simulink model "Robust_design_sinusoidal_validation"  (R2025b)
settings: Solver=VariableStepAuto  StartTime=0.0  StopTime=20  FixedStep=0.001  RelTol=1e-3
undefined symbols (not defined in the file): daq, degs2rpm, den, den_G, drv, Kxi, num, num_G, rdp, rpm2rads, sens, Ts, u_bar_max
settings Model: Creator=Enrico  LastModifiedBy=Enrico
settings DataIOCC: ReturnWorkspaceOutputsName=out_black_box

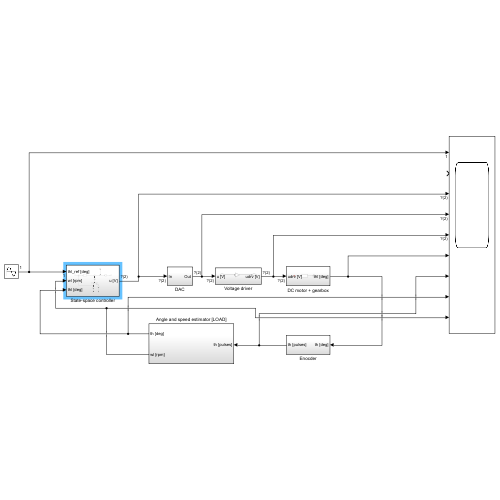
[thumbnail: Simulink's stored preview of the top-level diagram]
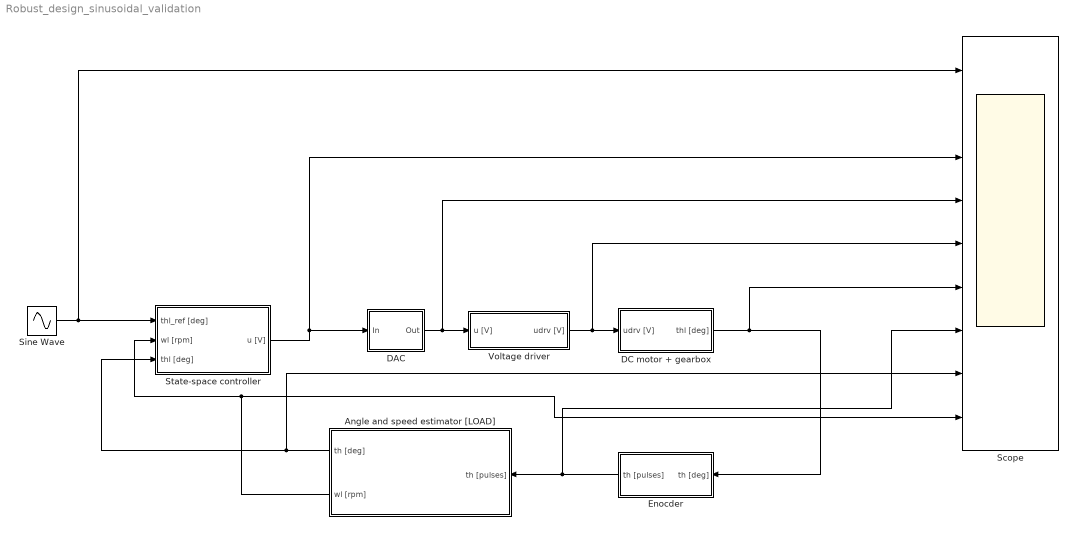
== system Robust_design_sinusoidal_validation ==
  Angle and speed estimator [LOAD] : Subsystem
  DAC : Subsystem
  DC motor + gearbox : Subsystem
  Enocder : Subsystem
  Scope : Scope  NumInputPorts=9
      settings: ActiveDisplayYMinimum=-1.2803910896593547  ActiveDisplayYMaximum=1.2800791059600789
  Sine Wave : Sin  Frequency=2*pi*0.5  SampleTime=0
  State-space controller : Subsystem
  Voltage driver : Subsystem
  wires:
  State-space controller/1(u [V]) -> Scope/3, DAC/1(In)
  DAC/1(Out) -> Scope/4, Voltage driver/1(u [V])
  Sine Wave/1 -> Scope/1, State-space controller/1(thl_ref [deg])
  Enocder/1(th [pulses]) -> Scope/7, Angle and speed estimator [LOAD]/1(th [pulses])
  Voltage driver/1(udrv [V]) -> Scope/5, DC motor + gearbox/1(udrv [V])
  DC motor + gearbox/1(thl [deg]) -> Scope/6, Enocder/1(th [deg])
  Angle and speed estimator [LOAD]/1(th [deg]) -> State-space controller/3(thl [deg]), Scope/8
  Angle and speed estimator [LOAD]/2(wl [rpm]) -> State-space controller/2(wl [rpm]), Scope/9

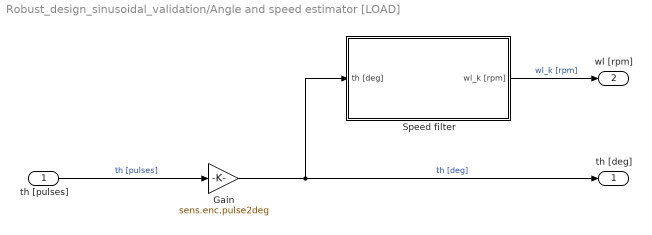
== system Robust_design_sinusoidal_validation/Angle and speed estimator [LOAD] ==
  th [pulses] : Inport
  Gain : Gain  Gain=sens.enc.pulse2deg
  Speed filter : Subsystem
  th [deg] : Outport
  wl [rpm] : Outport  Port=2
  wires:
  Speed filter/1(wl_k [rpm]) -> wl [rpm]/1  "wl_k [rpm]"
  th [pulses]/1 -> Gain/1  "th [pulses]"
  Gain/1 -> Speed filter/1(th [deg]), th [deg]/1  "th [deg]"

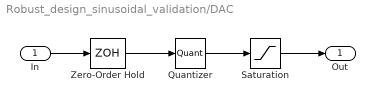
== system Robust_design_sinusoidal_validation/DAC ==
  In : Inport
  Quantizer : Quantizer  QuantizationInterval=daq.dac.q
  Saturation : Saturate  UpperLimit=daq.dac.fs  LowerLimit=-daq.dac.fs
  Zero-Order Hold : ZeroOrderHold  SampleTime=Ts
  Out : Outport
  wires:
  Quantizer/1 -> Saturation/1
  In/1 -> Zero-Order Hold/1
  Zero-Order Hold/1 -> Quantizer/1
  Saturation/1 -> Out/1

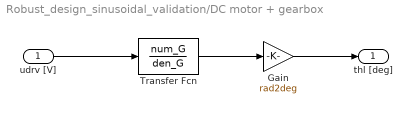
== system Robust_design_sinusoidal_validation/DC motor + gearbox ==
  udrv [V] : Inport
  Gain : Gain  Gain=rad2deg
  Transfer Fcn : TransferFcn  Numerator=num_G  Denominator=den_G
  thl [deg] : Outport
  wires:
  udrv [V]/1 -> Transfer Fcn/1
  Transfer Fcn/1 -> Gain/1
  Gain/1 -> thl [deg]/1

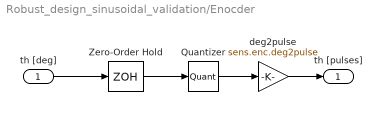
== system Robust_design_sinusoidal_validation/Enocder ==
  th [deg] : Inport
  Quantizer : Quantizer  QuantizationInterval=sens.enc.pulse2deg
  Zero-Order Hold : ZeroOrderHold  SampleTime=Ts
  deg2pulse : Gain  Gain=sens.enc.deg2pulse
  th [pulses] : Outport
  wires:
  Quantizer/1 -> deg2pulse/1
  th [deg]/1 -> Zero-Order Hold/1
  Zero-Order Hold/1 -> Quantizer/1
  deg2pulse/1 -> th [pulses]/1

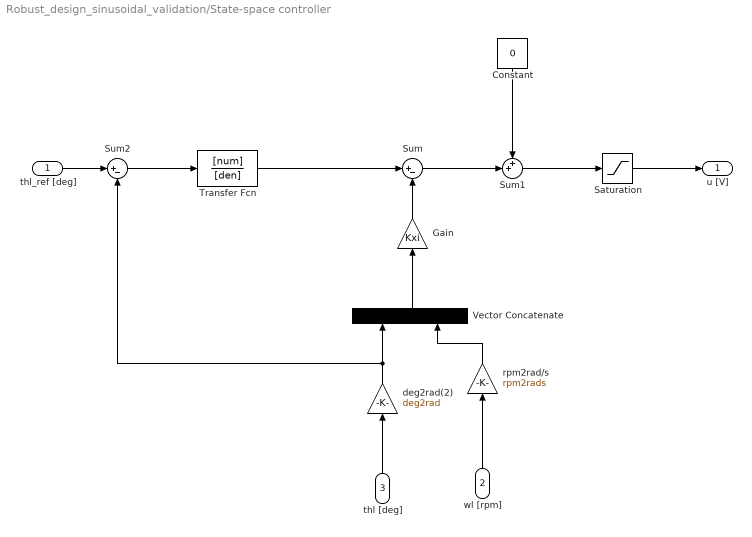
== system Robust_design_sinusoidal_validation/State-space controller ==
  thl_ref [deg] : Inport
  wl [rpm] : Inport  Port=2
  thl [deg] : Inport  Port=3
  Constant : Constant  Value=0
  Gain : Gain  Gain=Kxi
  Saturation : Saturate  UpperLimit=u_bar_max  LowerLimit=-u_bar_max
  Sum : Sum  Inputs=|+-
  Sum1 : Sum  Inputs=++|
  Sum2 : Sum  Inputs=|+-
  Transfer Fcn : TransferFcn  Numerator=[num]  Denominator=[den]
  Vector Concatenate : Concatenate
  deg2rad(2) : Gain  Gain=deg2rad
  rpm2rad/s : Gain  Gain=rpm2rads
  u [V] : Outport
  wires:
  Saturation/1 -> u [V]/1
  Sum/1 -> Sum1/2
  wl [rpm]/1 -> rpm2rad/s/1
  thl [deg]/1 -> deg2rad(2)/1
  deg2rad(2)/1 -> Sum2/2, Vector Concatenate/1
  rpm2rad/s/1 -> Vector Concatenate/2
  Vector Concatenate/1 -> Gain/1
  Gain/1 -> Sum/2
  Sum1/1 -> Saturation/1
  Sum2/1 -> Transfer Fcn/1
  thl_ref [deg]/1 -> Sum2/1
  Transfer Fcn/1 -> Sum/1
  Constant/1 -> Sum1/1

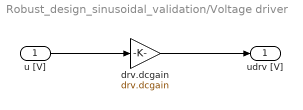
== system Robust_design_sinusoidal_validation/Voltage driver ==
  u [V] : Inport
  drv.dcgain : Gain  Gain=drv.dcgain
  udrv [V] : Outport
  wires:
  u [V]/1 -> drv.dcgain/1
  drv.dcgain/1 -> udrv [V]/1

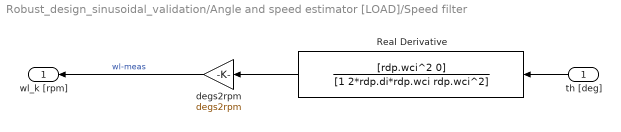
== system Robust_design_sinusoidal_validation/Angle and speed estimator [LOAD]/Speed filter ==
  th [deg] : Inport
  Real Derivative : TransferFcn  Numerator=[rdp.wci^2 0]  Denominator=[1 2*rdp.di*rdp.wci rdp.wci^2]
  degs2rpm : Gain  Gain=degs2rpm
  wl_k [rpm] : Outport
  wires:
  th [deg]/1 -> Real Derivative/1
  degs2rpm/1 -> wl_k [rpm]/1  "wl-meas"
  Real Derivative/1 -> degs2rpm/1
